simulink model "SOMANET"  (R2016b)
settings: Solver=VariableStepAuto  StartTime=0.0  StopTime=10.0  RelTol=1e-3
libraries: LibraryModel x1
settings Model: DataDictionary=ModelDictionary.sldd  Creator=Nathan  LastModifiedBy=Nathan

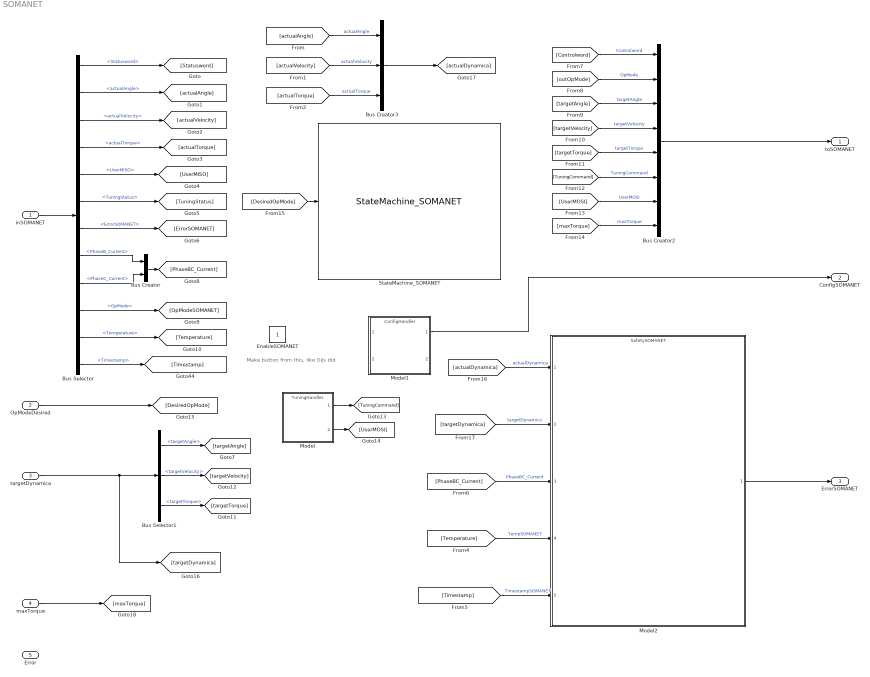
== system SOMANET ==
  note: Make button from this, like Gijs did
  inSOMANET : Inport  OutDataTypeStr=Bus: inSOMANET  BusOutputAsStruct=on
  OpModeDesired : Inport  Port=2
  targetDynamica : Inport  Port=3  OutDataTypeStr=Bus: targetDynamica  BusOutputAsStruct=on
  maxTorque : Inport  Port=4
  Error : Inport  Port=5
  Bus Creator : BusCreator  Inputs=2  OutDataTypeStr=Bus: PhaseBC_Current
  Bus Creator2 : BusCreator  Inputs=8
  Bus Creator3 : BusCreator  Inputs=3  OutDataTypeStr=Bus: actualDynamica  NonVirtualBus=on
  Bus Selector : BusSelector  OutputSignals=Statusword,actualAngle,actualVelocity,actualTorque,UserMISO,TuningStatus,ErrorSOMANET,PhaseB_Current,PhaseC_Current,OpMode,Temperature,Timestamp
  Bus Selector1 : BusSelector  OutputSignals=targetAngle,targetVelocity,targetTorque
  EnableSOMANET : Constant
      settings: OpenFcn=|
      | b = get_param(gcb,'value');
      | if (strcmp(b,'1')),
      |   set_param (gcb,'value','0');
      | else
      |   set_param(gcb,'value','1');
      | end;
  Model : ModelReference  ModelNameDialog=TuningHandler.slx  SimulationMode=Normal  ModelReferenceVersion=1.7
  Model1 : ModelReference  ModelNameDialog=ConfigHandler.slx  SimulationMode=Normal  ModelReferenceVersion=1.8
  Model2 : ModelReference  ModelNameDialog=SafetySOMANET.slx  SimulationMode=Normal  ModelReferenceVersion=1.19
  StateMachine_SOMANET : LibraryModel/StateMachine_SOMANET
  toSOMANET : Outport  OutDataTypeStr=Bus: toSOMANET  BusOutputAsStruct=on
  ConfigSOMANET : Outport  Port=2  OutDataTypeStr=Bus: ConfigSOMANET  BusOutputAsStruct=on
  ErrorSOMANET : Outport  Port=3
  wires:
  Model1/1 -> ConfigSOMANET/1
  inSOMANET/1 -> Bus Selector/1
  Bus Selector/1 -> [Statusword]  "<Statusword>"
  Bus Selector/2 -> [actualAngle]  "<actualAngle>"
  Bus Selector/3 -> [actualVelocity]  "<actualVelocity>"
  Bus Selector/4 -> [actualTorque]  "<actualTorque>"
  Bus Selector/5 -> [UserMISO]  "<UserMISO>"
  Bus Selector/6 -> [TuningStatus]  "<TuningStatus>"
  Bus Selector/7 -> [ErrorSOMANET]  "<ErrorSOMANET>"
  Bus Selector/8 -> Bus Creator/1  "<PhaseB_Current>"
  Bus Selector/10 -> [OpModeSOMANET]  "<OpMode>"
  Bus Selector/11 -> [Temperature]  "<Temperature>"
  Bus Selector/12 -> [Timestamp]  "<Timestamp>"
  Bus Selector/9 -> Bus Creator/2  "<PhaseC_Current>"
  Bus Creator/1 -> [PhaseBC_Current]
  [actualAngle] -> Bus Creator3/1  "actualAngle"
  [actualVelocity] -> Bus Creator3/2  "actualVelocity"
  [actualTorque] -> Bus Creator3/3  "actualTorque"
  [Temperature] -> Model2/4  "TempSOMANET"
  [Timestamp] -> Model2/5  "TimestampSOMANET"
  [PhaseBC_Current] -> Model2/3  "PhaseBC_Current"
  targetDynamica/1 -> [targetDynamica], Bus Selector1/1
  [Controlword] -> Bus Creator2/1  "Controlword"
  [outOpMode] -> Bus Creator2/2  "OpMode"
  [targetAngle] -> Bus Creator2/3  "targetAngle"
  [targetVelocity] -> Bus Creator2/4  "targetVelocity"
  [TuningCommand] -> Bus Creator2/6  "TuningCommand"
  [UserMOSI] -> Bus Creator2/7  "UserMOSI"
  [maxTorque] -> Bus Creator2/8  "maxTorque"
  [targetTorque] -> Bus Creator2/5  "targetTorque"
  Bus Creator2/1 -> toSOMANET/1
  Bus Selector1/3 -> [targetTorque]  "<targetTorque>"
  Bus Selector1/1 -> [targetAngle]  "<targetAngle>"
  Bus Selector1/2 -> [targetVelocity]  "<targetVelocity>"
  Model/1 -> [TuningCommand]
  Model/2 -> [UserMOSI]
  OpModeDesired/1 -> [DesiredOpMode]
  [DesiredOpMode] -> StateMachine_SOMANET/4
  Bus Creator3/1 -> [actualDynamica]
  [actualDynamica] -> Model2/1  "actualDynamica"
  [targetDynamica] -> Model2/2  "targetDynamics"
  maxTorque/1 -> [maxTorque]
  Model2/1 -> ErrorSOMANET/1
